simulink model "Two_cell_Fuzzy_BMS"  (R2024b)
settings: Solver=VariableStepAuto  StartTime=0.0  StopTime=100  RelTol=1e-3
undefined symbols (not defined in the file): Ion, Lithium
libraries: spsSeriesRLCBranchLib x6, spsIdealSwitchLib x4, spsMeanLib x4, spsCurrentMeasurementLib x3, spsBatteryLib x2, spsDiodeLib x2, spsMosfetLib x2, spsDCVoltageSourceLib x1, fuzblock x1, spsGroundLib x1, spsPWMGenerator2LevelLib x1, dspstat3 x1
settings Model: Creator=mridu  LastModifiedBy=Mridul
settings RTWCC: GPUComputeCapability=3.5

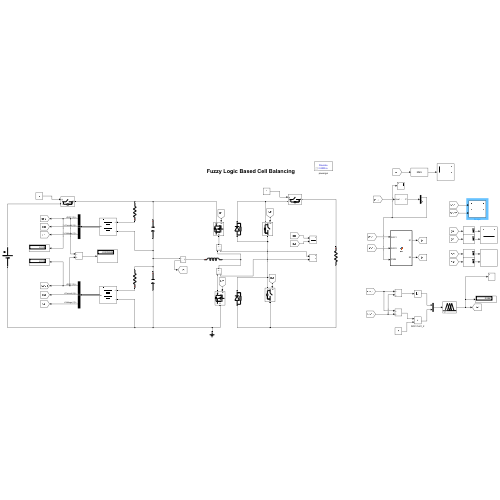
[thumbnail: Simulink's stored preview of the top-level diagram]
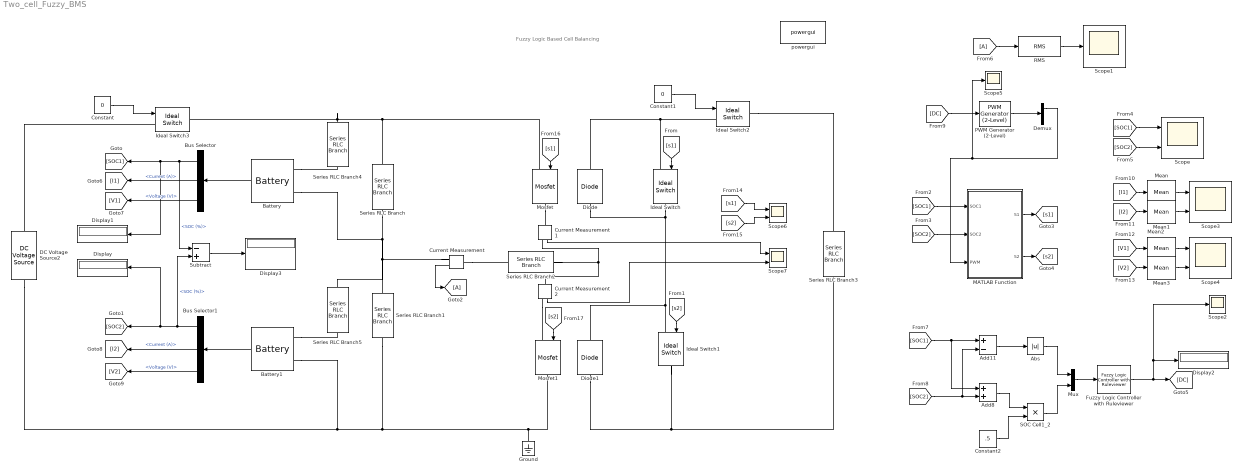
== system Two_cell_Fuzzy_BMS ==
  note: Fuzzy Logic Based Cell Balancing
  Abs : Abs  SaturateOnIntegerOverflow=off
  Add11 : Sum  Inputs=+-
  Add8 : Sum
  Battery : spsBatteryLib/Battery  BatType=Lithium-Ion  NomV=3.7  NomQ=3  SOC=70  Batt_Tr=0  PresetModel=on  MaxQ=3  MinV=2.775  FullV=4.3068  Dis_rate=1.3043  R=0.012333  Normal_OP=2.713  expZone="[3.9974     0.14739]"
  Battery1 : spsBatteryLib/Battery  BatType=Lithium-Ion  NomV=3.7  NomQ=3  SOC=60  Batt_Tr=0  PresetModel=on  MaxQ=3  MinV=2.775  FullV=4.3068  Dis_rate=1.3043  R=0.012333  Normal_OP=2.713  expZone="[3.9974     0.14739]"
  Bus Selector : BusSelector  OutputSignals=SOC (%),Current (A),Voltage (V)
  Bus Selector1 : BusSelector  OutputSignals=SOC (%),Current (A),Voltage (V)
  Constant : Constant  Value=0
  Constant1 : Constant  Value=0
  Constant2 : Constant  Value=.5
  Current Measurement : spsCurrentMeasurementLib/Current Measurement  PhasorSimulation=off  OutputType=Complex  PSBequivalent=0
  Current Measurement1 : spsCurrentMeasurementLib/Current Measurement  PhasorSimulation=off  OutputType=Complex  PSBequivalent=0
  Current Measurement2 : spsCurrentMeasurementLib/Current Measurement  PhasorSimulation=off  OutputType=Complex  PSBequivalent=0
  DC Voltage Source2 : spsDCVoltageSourceLib/DC Voltage Source  Amplitude=30  Measurements=None
  Demux : Demux  Outputs=2
  Diode : spsDiodeLib/Diode  Ron=0.001  Lon=0  Vf=0.8  IC=0  UseSnubber=0  Rs=500  Cs=250e-9  Measurements=off
  Diode1 : spsDiodeLib/Diode  Ron=0.001  Lon=0  Vf=0.8  IC=0  UseSnubber=0  Rs=500  Cs=250e-9  Measurements=off
  Display{,1..3} (4 alike) : Display
  From6 : From
  Fuzzy Logic Controller with Ruleviewer : fuzblock/Fuzzy Logic  Controller  with Ruleviewer  fismatrix=Cell_Balance1  Ts=2
  Goto2 : Goto
  Ground : spsGroundLib/Ground  LConnTagsString=a
  Ideal Switch{,1..3} (4 alike) : spsIdealSwitchLib/Ideal Switch  Ron=0.001  Lon=0  IC=0  Rs=1e5  Cs=inf  Measurements=off
  MATLAB Function : MATLAB Function  TreatAsAtomicUnit=on
  Mean{,1..3} (4 alike) : spsMeanLib/Mean  Freq=60  Vinit=0  Ts=0
  Mosfet : spsMosfetLib/Mosfet  Ron=0.1  Lon=0  Rd=0.01  Vfd=0  IC=0  Rs=1e5  Cs=inf  Measurements=off
  Mosfet1 : spsMosfetLib/Mosfet  Ron=0.1  Lon=0  Rd=0.01  Vfd=0  IC=0  Rs=1e5  Cs=inf  Measurements=off
  Mux : Mux  Inputs=2
  PWM Generator (2-Level) : spsPWMGenerator2LevelLib/PWM Generator (2-Level)  ModulatorType=Single-phase half-bridge (2 pulses)  ModulatorMode=Unsynchronized  Fc=500  Pc=0  nF=27  MinMax="[ -1  1 ]"  SamplingTechnique=Natural  ModulatingSignals=off  m=0.8  Freq=60  Phase=0  Ts=0  ShowCarrierOutport=off
  RMS : dspstat3/RMS  run=off  directionMode=Each column  dimension=1  InputProcessing=Columns as channels (frame based)  reset_popup=None
  SOC Cell1_2 : Product
  Scope{,3..4,6..7} (5 alike) : Scope  NumInputPorts=2
  Scope1 : Scope
  Scope2 : Scope
  Scope5 : Scope
  Series RLC Branch : spsSeriesRLCBranchLib/Series RLC Branch  LConnTagsString=__new0  RConnTagsString=__new0  BranchType=C  Resistance=1  Inductance=1e-3  SetiL0=off  InitialCurrent=0  Capacitance=1e-6  Setx0=off  InitialVoltage=0  Measurements=None
  Series RLC Branch1 : spsSeriesRLCBranchLib/Series RLC Branch  LConnTagsString=__new0  RConnTagsString=__new0  BranchType=C  Resistance=1  Inductance=1e-3  SetiL0=off  InitialCurrent=0  Capacitance=1e-6  Setx0=off  InitialVoltage=0  Measurements=None
  Series RLC Branch2 : spsSeriesRLCBranchLib/Series RLC Branch  LConnTagsString=__new0  RConnTagsString=__new0  BranchType=L  Resistance=1  Inductance=1e-3  SetiL0=off  InitialCurrent=0  Capacitance=1e-6  Setx0=off  InitialVoltage=0  Measurements=None
  Series RLC Branch3 : spsSeriesRLCBranchLib/Series RLC Branch  LConnTagsString=__new0  RConnTagsString=__new0  BranchType=R  Resistance=1  Inductance=1e-3  SetiL0=off  InitialCurrent=0  Capacitance=1e-6  Setx0=off  InitialVoltage=0  Measurements=None
  Series RLC Branch4 : spsSeriesRLCBranchLib/Series RLC Branch  LConnTagsString=__new0  RConnTagsString=__new0  BranchType=R  Resistance=0.01  Inductance=1e-3  SetiL0=off  InitialCurrent=0  Capacitance=1e-6  Setx0=off  InitialVoltage=0  Measurements=None
  Series RLC Branch5 : spsSeriesRLCBranchLib/Series RLC Branch  LConnTagsString=__new0  RConnTagsString=__new0  BranchType=R  Resistance=0.01  Inductance=1e-3  SetiL0=off  InitialCurrent=0  Capacitance=1e-6  Setx0=off  InitialVoltage=0  Measurements=None
  Subtract : Sum  Inputs=-+
  powergui : sps_lib/powergui  Priority=1  SimulationMode=Discrete  SampleTime=50e-5  frequency=60  Iterations=50  frequencyindice=0  Pbase=100e6  ErrMax=1e-4  UnitsV=kV  UnitsW=MW  buscounter=0  FunctionMessages=off  echomessages=off  EnableUseOfTLC=off  CurrentSourceSwitches=off  DisableSnubberDevices=off  DisableRonSwitches=off  DisableVfSwitches=off  DisplayEquations=off  AutomaticDiscreteSolvers=off  SolverType=Tustin/Backward Euler (TBE)  Interpol=off  ExternalGateDelay=off  methode=off  Ts=100  x0status=blocks  SPID=on  SwTol=0  HookPort=off  NonlinearTolerance=1e-4  nMaxIteration=100  ContinueOnMaxIteration=off  RestoreLinks=warning  ResistiveCurrentMeasurement=off  Frange=[0:2:500]  Ylog=off  Xlog=on  ShowGrid=off  save=off  variable=ZData  structure=0  ZoomFFT=off  StartTime=0.0  cycles=1  DisplayStyle=1  fundamental=60  FreqAxis=off  MaxFrequency=1000  frequencyindicesteady=1  RmsSteady=1  display=off
  wires:
  Battery/1 -> Bus Selector/1
  Battery1/1 -> Bus Selector1/1
  Constant/1 -> Ideal Switch3/1
  Constant1/1 -> Ideal Switch2/1
  Bus Selector1/1 -> Subtract/2, [SOC2], Display/1  "<SOC (%)>"
  Current Measurement/1 -> Goto2/1
  [s1] -> Ideal Switch/1
  [s2] -> Ideal Switch1/1
  MATLAB Function/2(S2) -> [s2]
  MATLAB Function/1(S1) -> [s1]
  [SOC1] -> MATLAB Function/1(SOC1)
  Demux/1 -> Scope5/1, MATLAB Function/3(PWM)
  [SOC2] -> MATLAB Function/2(SOC2)
  [DC] -> PWM Generator (2-Level)/1
  PWM Generator (2-Level)/1 -> Demux/1
  [SOC1] -> Scope/1
  [SOC2] -> Scope/2
  From6/1 -> RMS/1
  RMS/1 -> Scope1/1
  [SOC1] -> Add8/1, Add11/1
  [SOC2] -> Add11/2, Add8/2
  Add8/1 -> SOC Cell1_2/1
  Constant2/1 -> SOC Cell1_2/2
  Add11/1 -> Abs/1
  Abs/1 -> Mux/1
  SOC Cell1_2/1 -> Mux/2
  Mux/1 -> Fuzzy Logic Controller with Ruleviewer/1
  Fuzzy Logic Controller with Ruleviewer/1 -> [DC], Scope2/1, Display2/1
  Bus Selector/1 -> Subtract/1, [SOC1], Display1/1  "<SOC (%)>"
  Bus Selector/2 -> [I1]  "<Current (A)>"
  Bus Selector/3 -> [V1]  "<Voltage (V)>"
  Bus Selector1/2 -> [I2]  "<Current (A)>"
  Bus Selector1/3 -> [V2]  "<Voltage (V)>"
  Subtract/1 -> Display3/1
  [I1] -> Mean/1
  [I2] -> Mean1/1
  [V1] -> Mean2/1
  [V2] -> Mean3/1
  Mean/1 -> Scope3/1
  Mean1/1 -> Scope3/2
  Mean2/1 -> Scope4/1
  Mean3/1 -> Scope4/2
  [s1] -> Scope6/1
  [s2] -> Scope6/2
  [s1] -> Mosfet/1
  [s2] -> Mosfet1/1
  Current Measurement1/1 -> Scope7/1
  Current Measurement2/1 -> Scope7/2
  connections:
  Series RLC Branch/LConn1 -- Mosfet/LConn1 -- Series RLC Branch4/RConn1 -- Ideal Switch3/RConn1
  Ideal Switch3/LConn1 -- DC Voltage Source2/RConn1
  Diode1/LConn1 -- Ideal Switch1/RConn1 -- Series RLC Branch3/RConn1
  Ideal Switch2/RConn1 -- Series RLC Branch3/LConn1
  Series RLC Branch/RConn1 -- Current Measurement/RConn1 -- Series RLC Branch5/RConn1 -- Series RLC Branch1/LConn1 -- Battery/LConn2
  Ideal Switch/RConn1 -- Diode/LConn1 -- Diode1/RConn1 -- Ideal Switch1/LConn1
  Current Measurement/LConn1 -- Series RLC Branch2/LConn1
  Battery/LConn1 -- Series RLC Branch4/LConn1
  Battery1/LConn1 -- Series RLC Branch5/LConn1
  Series RLC Branch2/RConn1 -- Current Measurement2/LConn1 -- Current Measurement1/RConn1
  Ideal Switch2/LConn1 -- Diode/RConn1 -- Ideal Switch/LConn1
  DC Voltage Source2/LConn1 -- Battery1/LConn2 -- Series RLC Branch1/RConn1 -- Ground/LConn1 -- Mosfet1/RConn1
  Mosfet/RConn1 -- Current Measurement1/LConn1
  Current Measurement2/RConn1 -- Mosfet1/LConn1

== matlab function Two_cell_Fuzzy_BMS/MATLAB Function ==
  data: SOC1 input; S1 output; SOC2 input; PWM input; S2 output
function [S1, S2] = fcn(SOC1, SOC2, PWM)

if SOC2<SOC1
     S1=PWM;
     S2=0;
elseif SOC1<SOC2
     S1=0;
     S2=PWM;
else
     S1=0;
     S2=0;

end
